simulink model "EV_POWERTRAIN_Model"  (R2025a)
settings: Solver=VariableStepAuto  StartTime=0.0  StopTime=10.0  RelTol=1e-3
undefined symbols (not defined in the file or in its folder): Ion, Lithium
libraries: spsPWMGeneratorInterpolationLib x1, spsBatteryLib x1, spsPermanentMagnetSynchronousMachineLib x1, spsUniversalBridgeLib x1, sps_lib x1

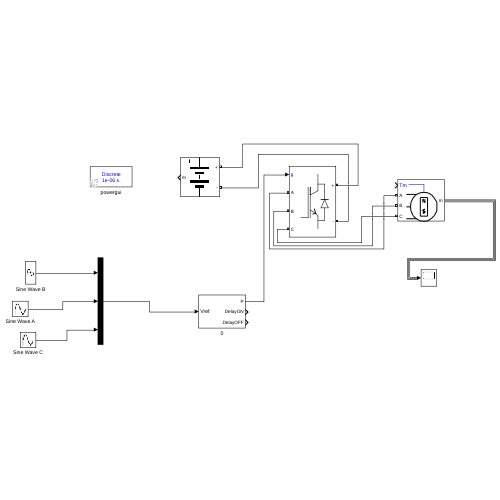
[thumbnail: Simulink's stored preview of the top-level diagram]
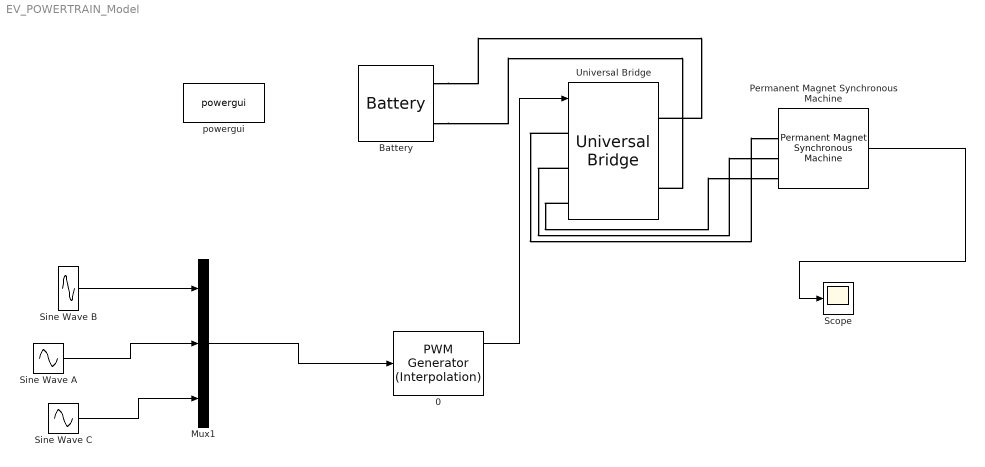
== system EV_POWERTRAIN_Model ==
  0 : spsPWMGeneratorInterpolationLib/PWM Generator (Interpolation)  GeneratorType=Two-level, three-phase  Fc=10000  InitialPhase=0  Ts=1e-6
      settings: LibrarySourceBlock=|
      | sps_lib/Power Electronics/Power Electronics Control/PWM Generator
      | (Interpolation)
  Battery : spsBatteryLib/Battery  BatType=Lithium-Ion  NomV=300  NomQ=100  SOC=80  Batt_Tr=0.01  PresetModel=on  MaxQ=100  MinV=225  FullV=349.1961  Dis_rate=43.4783  R=0.03  Normal_OP=90.4348  expZone="[324.1158      4.913043]"
  Mux1 : Mux  Inputs=3
  Permanent Magnet Synchronous Machine : spsPermanentMagnetSynchronousMachineLib/Permanent Magnet Synchronous Machine  NbPhases=3  FluxDistribution=Sinusoidal  RotorType=Round  MechanicalLoad=Torque Tm  PresetModel="03:  2.8 Nm 300 Vdc 4250 RPM - 3.2 Nm"  ShowDetailedParameters=on  MeasurementBus=on  Resistance=1.6  Inductance=8.5e-3  dqInductances=[8.5e-3,8.5e-3]  La=0.006365  MachineConstant=Flux linkage established by magnets (V.s)  Flux=0.1852  VoltageCst=67.1831  TorqueCst=0.5556  Flat=120  Mechanical=[0.0001854 5.396e-05 2 0]  PolePairs=2  InitialConditions=[0,0, 0,0]  InitialConditions5ph=[0 0 0 0 0 0]  RefAngle=90 degrees behind phase A axis (modified Park)  IterativeDiscreteModel=Trapezoidal non iterative  TsBlock=-1  TsPowergui=0
  Scope : Scope
      settings: ActiveDisplayYMinimum=-1794.1120554617908  ActiveDisplayYMaximum=439.42605918449283
  Sine Wave A : Sin  Frequency=2*pi*50  SampleTime=0
  Sine Wave B : Sin  Frequency=2*pi*50  Phase=-120*pi/180  SampleTime=0
  Sine Wave C : Sin  Frequency=2*pi*50  Phase=120*pi/180  SampleTime=0
  Universal Bridge : spsUniversalBridgeLib/Universal Bridge  Arms=3  SnubberResistance=1e6  SnubberCapacitance=inf  Device=IGBT / Diodes  Ron=1e-3  Lon=0  ForwardVoltages="[  0  0  ]"  ForwardVoltage=0  GTOparameters=[ 10e-6 , 20e-6 ]  IGBTparameters=[ 1e-6 , 2e-6 ]  Measurements=All voltages and currents  Measurements_2=None  converterType=Rectifier
  powergui : sps_lib/powergui  Priority=1  SimulationMode=Discrete  SampleTime=1e-6  frequency=60  Iterations=50  frequencyindice=0  Pbase=100e6  ErrMax=1e-4  UnitsV=kV  UnitsW=MW  buscounter=0  FunctionMessages=off  echomessages=off  EnableUseOfTLC=off  CurrentSourceSwitches=off  DisableSnubberDevices=off  DisableRonSwitches=off  DisableVfSwitches=off  DisplayEquations=off  AutomaticDiscreteSolvers=off  SolverType=Tustin/Backward Euler (TBE)  Interpol=off  ExternalGateDelay=off  methode=off  Ts=100  x0status=blocks  SPID=on  SwTol=0  HookPort=off  NonlinearTolerance=1e-4  nMaxIteration=100  ContinueOnMaxIteration=off  RestoreLinks=warning  ResistiveCurrentMeasurement=off  Frange=[0:2:500]  Ylog=off  Xlog=on  ShowGrid=off  save=off  variable=ZData  structure=0  ZoomFFT=off  StartTime=0.0  cycles=1  DisplayStyle=1  fundamental=60  FreqAxis=off  MaxFrequency=1000  frequencyindicesteady=1  RmsSteady=1  display=off
  wires:
  Sine Wave B/1 -> Mux1/1
  Sine Wave A/1 -> Mux1/2
  Sine Wave C/1 -> Mux1/3
  Mux1/1 -> 0/1
  0/1 -> Universal Bridge/1
  Permanent Magnet Synchronous Machine/1 -> Scope/1
  connections:
  Universal Bridge/LConn1 -- Permanent Magnet Synchronous Machine/LConn1
  Universal Bridge/LConn2 -- Permanent Magnet Synchronous Machine/LConn2
  Universal Bridge/LConn3 -- Permanent Magnet Synchronous Machine/LConn3
  Battery/LConn2 -- Universal Bridge/RConn2
  Battery/LConn1 -- Universal Bridge/RConn1
